simulink library "simetranss"  (R2024b)
settings: Solver=VariableStepAuto  StartTime=0.0  StopTime=10.0  RelTol=1e-3
PostLoadFcn:
  | Ts=1e-6
InitFcn:
  | Ts=1e-6
undefined symbols (not defined in the file): C, C_601, C_603, C_606, CC, Csnu, Csnubber, DiscIntNeverNeededParam, DPL, DPL1ph, FluxTable, ft2km, gcbh, h, Half, Imap2, L, L_601, L_603, L_606, Lbase, LpejoSw, Newton, R_601, R_603, R_606, Raphson, ResistanceM, Roff, Ron, RotorAngles, Rsnu, Rsnubber, Rt4, SampleTime, simetran, sps, sps_rtmsupport, StatorCurrents, T_2wind_ratio, T_Lpu, T_Lpu_pri, T_Rpu, T_Rpu_pri, T_Vpri, T_Vpri_15comp, T_Vsec, Ti, Ts_Power, Z, Zbase, Zm
libraries: fl_lib x248, ee_lib x146, nesl_utility x122, $bdroot x29, simulink x15, eeGeneralControl x2, spsStairGeneratorLib x2, artemis x1
(part 3 of 12)

== system simetranss/Network decoupling ==
  note: DC bus decoupling blocks
  DCbus Vrecv : Subsystem  mask(DC Bus decoupling (Receiving-V)){Ts=Ts}
      mask prompts: Ts "Sample time (s)"
      mask help: This block is used to create a delay in DC-busses..
      mask Display: disp('Vcap recv')
  DCbus Vsend : Subsystem  mask(DC Bus decoupling (Sending-V)){Ts=Ts}
      mask prompts: Ts "Sample time (s)"
      mask help: This block is used to create a delay in DC-busses.
      mask Display: disp('Vcap send')
  MATE 3-phase Compensated Half-Stubline : Subsystem  mask(MATE 3-phase Compensated Stubline){stype=3-phase line without couplings, FF=60, RR=R_601, LL=L_601, CC=C_601, len=2000*ft2km, Ts=Ts, comp=on, stdel=off}
      mask prompts: stype "Stubline type"; FF "Nominal frequency (Hz)"; RR "Resistance (Ohms/km)"; LL "Inductance (H/km)"; CC "Capacitance (F/km)"; len "Length (km)"; Ts "Sample time (s)"; comp "Compensate reactive power on this half of the stubline"; stdel "Concurrent simulation: remove internal stubline delay"
      mask help:
      | This block Implements a 3-phase stubline with reactive power compensation.
      |
      |
      | The block has 3 main options:
      | -uncoupled 3-phase
      | -single-mode coupled 3-phase
      | - dual-mode coupled 3-phase
      |
      | In single-mode, the stubline implements Bergeron line model with losses having the same 1-step propagation delay for all 3 modes. In the dual-mode option, the gound mode has a exact 2-step delay (main mode still has a 1 step-delay).The advantage of coupled modes is that some inter-phase capacitance is included in the stubline, therefore requirinf less overall reactive compensation.
      |
      | Line reactive compensation can only be made on only ONE of the two half stubline.
      |
      | Concurrent simulation: remove internal stubline delay : when using Simulink Concurrent simulation option, selecting this option removes the model 1/z communication delay, which is replaced implicitely by the concurrent simulation delay.
      mask init:
      | % Get current block
      | currentBlock = gcb;
      | 
      | dee=get_param(currentBlock,'stdel');
      | if isequal(dee,'on')
      |     set_param([currentBlock '/stubline/halfstub/zz'],'Commented','through');
      | else
      |     set_param([currentBlock '/stubline/halfstub/zz'],'Commented','off');
      | end
      | 
      | %Ts=2.5e-5;
      | % C1= (Ts)^2/L1;
      | Length=1;
      | Phases=3;
      | Frequency=FF;
      | Rabc = RR*len;
      | Labc = LL*len;
      | Cabc = CC*len;
      | 
      | Lm_abc_min = min(min(Labc));
      | Ls_abc_min = min(diag(Labc));
      | Lm_abc_max = max(max(Labc-diag(diag(Labc))));
      | 
      | Rm_abc_min = min(min(Rabc));
      | Rs_abc_min = min(diag(Rabc));
      | Rm_abc_max = max(max(Rabc-diag(diag(Rabc))));
      | 
      | Step = Ls_abc_min/10;
      | StepR = Rs_abc_min/10;
      | 
      | % xqnum=str2num(get_param(currentBlock,'xq'));
      | % x=xqnum(1);
      | % q=xqnum(2);
      | sel=0; % default delays all equal.
      | Ti=[1/sqrt(3) 1/sqrt(2)  1/sqrt(6); 1/sqrt(3) -1/sqrt(2)  1/sqrt(6); 1/sqrt(3) 0 -sqrt(2/3)];
      | st=get_param(currentBlock,'stype');
      | 
      | if isequal (st, '3-phase coupled line (1 mode)')
      |     %x=3
      |     %============== corrected code =====
      |     x=3;y=4;
      |     %===================================
      |     Lm = Lm_abc_min;
      |     L1 = 2*Lm;      %changed (is was L1 = 3*Lm;)
      |     Inductance = [x 1 1;1 x 1; 1 1 x]*L1/(x-1);
      |     L_diff = Labc - Inductance;
      | 
      |     Rm = Rm_abc_min;
      |     R1 = 2*Rm;      %changed (is was R1 = 3*Rm;)
      |     Resistance = [x 1 1;1 x 1; 1 1 x]*R1/(x-1);
      |     R_diff = Rabc - Resistance;
      | 
      | 
      |     if Ls_abc_min - 4*Lm - Step < Lm_abc_max - Lm
      |         Lm = (Ls_abc_min - Lm_abc_max - Step)/2;
      |         L1 = 2*Lm;      %changed (is was L1 = 3*Lm;)
      |         Inductance = [x 1 1;1 x 1; 1 1 x]*L1/(x-1);
      |         L_diff = Labc - Inductance;
      | 
      |         Rm = (Rs_abc_min - Rm_abc_max - StepR)/2;
      |         R1 = 2*Rm;      %changed (is was R1 = 3*Rm;)
      |         Resistance = [x 1 1;1 x 1; 1 1 x]*R1/(x-1);
      |         R_diff = Rabc - Resistance;
      |     end
      |     
      |     %=============== corrected code for capacitance =================
      |     C1 = Ts^2/L1;
      |     Capacitance =[y -1 -1;-1 y -1; -1 -1 y]*C1/(y+1);
      |     %==================================================================
      |     
      | 
      | elseif isequal(st,'3-phase coupled line (2 modes)')
      |     q=0.5;
      |     Lm = Lm_abc_min;
      |     L1 = Lm;
      |     Inductance = [1 q q; q 1 q; q q 1]*L1/(1-q);
      |     L_diff = Labc - Inductance; 
      | 
      |     R1 = Rm_abc_min ;
      |     Resistance = [1 q q; q 1 q; q q 1]*R1/(1-q);
      |     R_diff = Rabc - Resistance;
      | 
      |     Step = Ls_abc_min/10;
      |     StepR = Rs_abc_min/10;
      | 
      |     if Ls_abc_min - 2*Lm - Step < Lm_abc_max - Lm                                              
      |         Lm = Ls_abc_min - Lm_abc_max - Step;
      |         L1 = Lm;
      |         Inductance = [1 q q; q 1 q; q q 1]*L1/(1-q);
      |         L_diff = Labc - Inductance;
      | 
      |         R1 = Rs_abc_min - Rm_abc_max - StepR;
      |         Resistance = [1 q q; q 1 q; q q 1]*R1/(1-q);
      |         R_diff = Rabc - Resistance;
      |     end
      | 
      |     C1 = Ts^2/L1;
      |     Capacitance = eye(3)*C1; 
      |     
      | 
      | sel=1;  % with 2 mode case, mode 0 is 2 time slower!
      | 
      | elseif isequal(st,'3-phase line without couplings')
      |     L1 = Ls_abc_min - Lm_abc_max - Step;
      |     Inductance = eye(3)*L1;
      |     L_diff = Labc - Inductance;
      | 
      |     R1 = Rs_abc_min - Rm_abc_max - StepR;
      |     Resistance = eye(3)*R1;
      |     R_diff = Rabc - Resistance;
      |     C1 = Ts^2/L1;
      |     Capacitance = eye(3)*C1;   
      | else
      |     error('stubline type not found')
      | end
      | 
      | C_diff = Cabc;
      | 
      | % % Get electric variables
      | 
      | %============= These two lines should be removed ======
      | % C1 = Ts^2/L1
      | % Capacitance = eye(3)*C1;
      | %======================================================
      | 
      | [Zm,R,v,Ti,to,Rt4,h,Zimp,Zmat,Yphase,ResistanceM] = ssc_dpl_cb(currentBlock,'variable_mask_maskinitialization', Phases, Frequency, Resistance, Inductance, Capacitance, Length);
      | 
      | verif=sum(to/Ts);
      | if (2.99999<verif && verif<3.00001) || (3.99999<verif && verif<4.00001)
      |     % sum of delays should be 3 or 4
      | else
      |     error(['The stubline block ' gcb ' computed a non-integer propagation delay.']);
      | end
      | 
      | if isequal(st,'3-phase line without couplings')
      |     for i=1:3
      |         for j=1:3
      |             if i~=j  && ResistanceM(i,j)<0
      |                 ResistanceM(i,j)=1e10;   
      |             end
      |         end
      |     end
      | end
      | 
      | 
      | % % Compute Compensation block parameters
      | 
      | % Disabled here
      | 
      | L_comp=1/((2*pi*FF)^2*C1);     % calculate compensating inductance
      | R_damp=1e8;                     % set damping resistance to high value
      | C_damp=1e-8;                   % set coupling capacitor to low value
      mask TypeOptions stype: 3-phase coupled line (1 mode) | 3-phase coupled line (2 modes) | 3-phase line without couplings
      mask Callback comp:
      | block=gcb;
      | st=get_param(block,'comp');
      | if isequal(st,'on')
      |     set_param([block '/Compensate'], 'Commented', 'off');
      |     set_param([block '/Pass'], 'Commented', 'on');
      | else
      |     set_param([block '/Compensate'], 'Commented', 'on');
      |     set_param([block '/Pass'], 'Commented', 'off');
      | end
      mask Display:
      | plot(0,0,100,100,[20,20,40,40,60,40,40,20,20,10]+10,[50,40,40,50,50,50,61,61,50,50],[23 32 23 32]+10,[52,52,42,42],[33 35]+10,[55 55],[37 37]+10,[57 53])
      | 
      | %disp([ 32 32 'Full STUB'])
  RTScapeHalfStub : Subsystem  mask(SimScape Stubline){Phases=2 with differential inputs, pu=on, L=100e-3, Lpu=0.03, R=0.05, Rpu=0.02, S_base=1e5, V_base=1000, F_base=60, Ts=Ts}
      mask prompts: Phases "Number of phases N"; pu "Per-Unit value specification"; L "Inductance (H)"; Lpu "Inductance (pu)"; R "Resistance (Ohms)"; Rpu "Resistance (pu)"; S_base "Nominal Power (VA)"; V_base "Nominal voltage (V)"; F_base "Nominal frequency (Hz)"; Ts "Sample time (s)"
      mask help:
      | The simScape Stubline block implements a single distributed parameters transmission line model with exactly one time step propagation delay. It is optimized for real-time simulation.
      |
      | The SimScape Stubline block permits the decoupling of state-space system equations of networks on both sides of the stubline.
      mask init:
      | currentBlock = gcb;
      | 
      | 
      | 
      | % if isempty(S_base*V_base*F_base*Ts) 
      | %     return
      | % end
      | 
      | % Calculate Per Units
      | 
      | I_base=S_base/V_base;
      | w_base=2*pi*F_base;
      | Z_base=V_base/I_base;
      | L_base=Z_base/w_base;
      | C_base=1/(Z_base*w_base);
      | if pu == 1
      |     L=Lpu*L_base;
      |     R=Rpu*Z_base;
      | end
      | C = (Ts)^2/L;
      | Cpu = C / C_base;
      | 
      | 
      | 
      | 
      | 
      | 
      | % Calculate internal variables
      | [C, Zm, Rt4, h, w1, Z] = stub_cb(currentBlock,'lick it', 1, L, R, Ts);
      mask Help: eval('fts2help(''stubline'');');
      mask TypeOptions Phases: 1 | 2 | 3 | 4 | 5 | 6 | 2 with differential inputs
      mask Callback pu:
      | % Set mask display
      | stub_cb(gcb,'maskinitialization',1);
      mask Display: disp(sprintf('Half stubline\nL=  %s  mH\nC=  %s  uF\nR=  %s \\Omega',num2str(L*1e3,4), num2str(C*1e6,4), num2str(R,4)),'texmode','on');
  Seven-winding Decoupling Transformer : Subsystem  Tag=PublishSubsystem  mask(MATE 7-winding stubline transformer){Vpri=T_Vpri/sqrt(3), RLpri=[T_Rpu_pri*Zbase T_Lpu_pri*Lbase], Vwdn=[ T_Vsec/sqrt(3) T_Vsec T_Vsec/sqrt(3)*T_Vpri_15comp T_Vsec/sqrt(3)*T_2wind_ratio*T_Vpri_15comp T_Vsec/sqrt(3)*T_Vpri_15comp T_Vsec/sqrt(3)*T_2wind_ratio*T_Vpri_15comp  ], Lwdn=[T_Lpu_pri   T_Lpu T_Lpu T_Lpu*T_Vpri_15comp  T_Lpu*T_2wind_ratio*T_Vpri_15comp T_Lpu*T_Vpri_15comp  T_Lpu*T_2wind_ratio*T_Vpri_15comp ]*Lbase, Rwdn=[     T_Rpu            T_Rpu    T_Rpu*T_Vpri_15comp T_Rpu*T_2wind_ratio*T_Vpri_15comp T_Rpu*T_Vpri_15comp T_Rpu*T_2wind_ratio*T_Vpri_15comp]*Zbase, Rearth=1e6, Ts=Ts}
      mask prompts: Vpri "Primary voltage (V)"; RLpri "Primary winding resistance (Ohms) and leakaege inductance (H)"; Vwdn "Secondary winding voltages"; Lwdn "Secondary winding leakeage inductance (H)"; Rwdn "Secondary winding resistance (Ohms)"; Rearth "Secondary resistance to earth (Ohms)"; Ts "Sample time (s)"
      mask help: This is a stubline transformer in which all secondary windings are decoupled with a 1 step-delay transmission line (stubline).
  Three-Phase 2-Windings Decoupling Transformer : Subsystem  mask(MATE Decoupling Three-Phase Transformer (Two Windings)){deconf=Complete transformer, stdel=off, Winding1Connection=Yn, Winding2Connection=Yn, UNITS=pu, NominalPower=[ 500e3 , 60 ], Winding1=[ 4160 , 0.001 , 0.01 ], Winding2=[ 480, 0.01 , 0.01 ], Rm=500, Lm=500}
      mask prompts: deconf "Decoupling configuration"; stdel "Concurrent simulation: remove internal stubline delay"; Winding1Connection "Primary connection (ABC terminals):"; Winding2Connection "Secondary connection (abc terminals):"; NominalPower "Nominal power and frequency  [ Pn(VA) , fn(Hz) ]"; Winding1 "Winding 1 parameters [ V1 Ph-Ph(Vrms) , R1(pu) , L1(pu) ]"; Winding2 "Winding 2 parameters [ V2 Ph-Ph(Vrms) , R2(pu) , L2(pu) ]"; Rm "Magnetization resistance  Rm (pu)"; Lm "Magnetization inductance  Lm (pu)"
      mask help:
      | This block implements a  decoupling three-phase transformer.
      | The secondary winding leakeage inductance and resistance are implemented as stublines.
      | Only Y-Y with accesible neutral is available for now.
      mask init:
      | block = gcb;
      | dee=get_param(block,'stdel');
      | if isequal(dee,'on')
      |     set_param([block '/del1'],'Commented','through');
      |     set_param([block '/del2'],'Commented','through');
      |     set_param([block '/del3'],'Commented','through');
      |     set_param([block '/del4'],'Commented','through');
      | else
      |     set_param([block '/del1'],'Commented','off');
      |     set_param([block '/del2'],'Commented','off');
      |     set_param([block '/del3'],'Commented','off');
      |     set_param([block '/del4'],'Commented','off');
      | end
      | 
      | m=ThreePhaseTransformersPU(block);
      | 
      | block = gcb;
      | str=get_param(block,'deconf');
      | if isequal(str,'Complete transformer')
      |     set_param([block '/pri'], 'Commented', 'off');
      |     set_param([block '/sec'], 'Commented', 'off');
      |     set_param([block '/path'], 'Value', '1');
      |     replace_block (block ,'Followlinks' ,'on' ,'Name' ,'houtsec' ,'BlockType' ,'Outport' ,'Terminator' ,'noprompt' );
      |     replace_block (block ,'Followlinks' ,'on' ,'Name' ,'houtpri' ,'BlockType' ,'Outport' ,'Terminator' ,'noprompt' );
      |     replace_block (block ,'Followlinks' ,'on' ,'Name' ,'hinsec' ,'BlockType' ,'Inport' ,'Ground' ,'noprompt' );
      |     replace_block (block ,'Followlinks' ,'on' ,'Name' ,'hinpri' ,'BlockType' ,'Inport' ,'Ground' ,'noprompt' );
      |     MATE_xfo_ports(block, 'addABC');
      |     MATE_xfo_ports(block, 'addN');
      |     MATE_xfo_ports(block, 'addabc');
      |     MATE_xfo_ports(block, 'addn');
      | elseif isequal(str,'Primary side')
      |     set_param([block '/pri'], 'Commented', 'off');
      |     set_param([block '/sec'], 'Commented', 'on');
      |     set_param([block '/path'], 'Value', '0');
      |     try
      |     replace_block (block ,'Followlinks' ,'on' ,'Name' ,'houtsec' ,'BlockType' ,'Outport' ,'Terminator' ,'noprompt' );
      |     replace_block (block ,'Followlinks' ,'on' ,'Name' ,'houtpri' ,'BlockType' ,'Terminator','Outport' ,'noprompt' );
      |     replace_block (block ,'Followlinks' ,'on' ,'Name' ,'hinsec' ,'BlockType' ,'Inport' ,'Ground' ,'noprompt' );
      |     replace_block (block ,'Followlinks' ,'on' ,'Name' ,'hinpri' ,'BlockType' ,'Ground' ,'Inport' ,'noprompt' );
      |     catch
      |         warning('possible port error on Primary')
      |     end
      |     MATE_xfo_ports(block, 'addABC');
      |     MATE_xfo_ports(block, 'addN');
      |     MATE_xfo_ports(block, 'removeabc');
      |     MATE_xfo_ports(block, 'removen');
      | elseif isequal(str,'Secondary side')
      |     set_param([block '/pri'], 'Commented', 'on');
      |     set_param([block '/sec'], 'Commented', 'off');
      |     set_param([block '/path'], 'Value', '0');
      |     try
      |     replace_block (block ,'Followlinks' ,'on' ,'Name' ,'houtsec' ,'BlockType' ,'Terminator','Outport' ,'noprompt' );
      |     replace_block (block ,'Followlinks' ,'on' ,'Name' ,'houtpri' ,'BlockType' ,'Outport' ,'Terminator','noprompt' );
      |     replace_block (block ,'Followlinks' ,'on' ,'Name' ,'hinsec' ,'BlockType' , 'Ground' ,'Inport','noprompt' );
      |     replace_block (block ,'Followlinks' ,'on' ,'Name' ,'hinpri' ,'BlockType' ,'Inport' ,'Ground' ,'noprompt' );
      |     catch
      |         warning('possible port error on Secondary')
      |     end
      |     MATE_xfo_ports(block, 'removeABC');
      |     MATE_xfo_ports(block, 'removeN');
      |     MATE_xfo_ports(block, 'addabc');
      |     MATE_xfo_ports(block, 'addn');
      | else 
      |     error('Option not reckognized!')
      | end
      mask TypeOptions deconf: Complete transformer | Primary side | Secondary side
      mask TypeOptions Winding1Connection: Y | Yn | Yg | Delta (D1) | Delta (D11)
      mask TypeOptions Winding2Connection: Y | Yn | Yg | Delta (D1) | Delta (D11)
      mask TypeOptions UNITS: SI | pu
      mask DialogControl ParameterTabVar0 Prompt: Configuration
      mask DialogControl ParameterTabVar01 Prompt: Parameters
      mask Display:
      | plot(-180,-220,180,220,[-100,-40],[0,0],[100,40],[0,0],[2 42 74 94 100 90 66 30 0 2 42 74 94 100 90 66 30 0 2 42 74 94 100 90 66 30 0 2 42 74 94 100 90 66 30 0]*.4-55,[-45 -45 -34 -17 3 22 38 48 50 50 55 66 83 103 122 138 148 150 150 155 166 183 203 222 238 248 250 250 255 266 283 303 322 338 348 348]*0.5-75,[2 42 74 94 100 90 66 30 0 2 42 74 94 100 90 66 30 0 2 42 74 94 100 90 66 30 0 2 42 74 94 100 90 66 30 0]*-.4+55,[-45 -45 -34 -17 3 22 38 48 50 50 55 66 83 103 122 138 148 150 150 155 166 183 203 222 238 248 250 250 255 266 283 303 322 338 348 348]*0.5-75)
      | %plot(-180,-220,180,220,[-100,-40]*-1,[0,0],[2 42 74 94 100 90 66 30 0 2 42 74 94 100 90 66 30 0 2 42 74 94 100 90 66 30 0 2 42 74 94 100 90 66 30 0]*.4-55,[-45 -45 -34 -17 3 22 38 48 50 50 55 66 83 103 122 138 148 150 150 155 166 183 203 222 238 248 250 250 255 266 283 303 322 338 348 348]*-0.5+75)
      | 
      | disp(['Y   Y'  10 10 10 10 10 'z-1'])
  wires:
  DCbus Vsend/1(Vc) -> DCbus Vrecv/1(Vc-z)
  DCbus Vrecv/1(Idc) -> DCbus Vsend/1(Iin)

== system simetranss/Passive ==
  MATE Single-Phase Load : Subsystem  mask(MATE 1-phase load){Vabc=300, Fn=60, typ=Series RL, Pabc=[160 ]*1e3, QLabc=[ 90]*1e3, QCabc=[190  ]*1e3}
      mask prompts: Vabc "Nominal phase-to-ground voltage (Vrms)"; Fn "Nominal frequency fn (Hz):"; typ "Load type"; Pabc "Active powers (W)"; QLabc "Inductive reactive powers (positive var):"; QCabc "Capacitive reactive powers (positive var):"
      mask help: This block implements either a series RL load or a purely capacitive load.
      mask init:
      | block=gcb;
      | type=get_param(block,'typ');
      | 
      | if isequal (type,'Series RL')
      | j=sqrt(-1);
      | S=Pabc-j*QLabc;
      | Z=Vabc.*Vabc./S;
      | R=real(Z);
      | L=imag(Z)/2/pi/Fn;
      | 
      | s1 = 0;
      | s2 =-50;
      | s3 = 450;
      | s4 =50;
      | r1 = [0    30    30    38    53    68    83    98   113   120   120   150];
      | r2 =[0     0     0    25   -25    25   -25    25   -25     0     0     0];
      | c1 =[0];
      | c2 =[0 ];
      | c3 =[0];
      | c4 = [0];
      | c5=0;
      | c6=0;
      | l1 =[150   173   173   174   178   184   190   197   202   205   206   204   201 201   197   196   198   201   207   214   220   225   229   229   227   224   224   220   219   221   225   230   237   243   249   252   253   251   247  247   244   243   244   248   254   260   267   272   275   276   276   300 450];
      | l2 =[0     0     1    11    19    24    25    23    17     8    -2   -12   -18 -18    -9     1    11    19    24    25    23    17     8    -2   -12   -18 -18    -9     1    11    19    24    25    23    17     8    -2   -12   -18  -18    -9     1    11    19    24    25    23    17     8     0     0     0 0];
      | sca=0.5;
      | neutral=0;
      | ground=1;
      | else
      |     j=sqrt(-1);
      | S=QCabc;
      | Z=Vabc.*Vabc./S;
      | w=2*pi*Fn;
      | % Z=1/(wC)
      | C=1/w./Z;
      | 
      | 
      | s1 = 0;
      | s2 =-50;
      | s3 = 450;
      | s4 =50;
      | r1 = [0    ];
      | r2 =[0   ];
      | c1 =[450   390   390   393   395   393   390   390   393   395]-200;
      | c2 =[0     0     8    16    25    16     8    -8   -16   -25];
      | c3 =[360   360   360   250]-200;
      | c4 = [25   -25     0     0];
      | c5 =[ 455 200];
      | c6 = [0 0];
      | l1 =[0];
      | l2 =[0 ];
      | sca=0.5;
      | neutral=0;
      | 
      | ground=1;
      | 
      | 
      | 
      | end
      mask TypeOptions typ: Series RL | Capacitance
      mask Callback typ:
      | block = gcb;
      | type=get_param(block,'typ');
      | 
      | visib=get_param(block,'MaskVisibilities');
      | if isequal(type,'Series RL')
      |     visib{4}='on';;visib{5}='on';visib{6}='off';
      | else
      |     visib{4}='off';visib{5}='off';visib{6}='on';
      | end
      | set_param(block,'MaskVisibilities',visib);
      | 
      | 
      | if isequal(type,'Series RL')
      |     set_param([block '/RLseries'], 'Commented', 'off');
      |     set_param([block '/C'], 'Commented', 'on');
      | else
      |     set_param([block '/RLseries'], 'Commented', 'on');
      |     set_param([block '/C'], 'Commented', 'off');
      | end
      mask Display:
      | plot(s1-160,s2,s3+80,s4,r1,r2,l1,l2,c1,c2,c3,c4,c5,c6)
      | 
      | plot( ground*[s3,s3], ground*[-s2/4,s2/4])
      | plot( ground*[s3+30,s3+30], ground*[-s2/6,s2/6])
      | plot( ground*[s3+60,s3+60], ground*[-s2/10,s2/10])
      | 
      | plot( neutral*[s3,s3+80], neutral*[0,0])
  MATE Unbalanced Load : Subsystem  AncestorBlock=simetran/SimScape RL Load3  mask(MATE  3-phase unbalanced load){Vabc=[ 0.993926 1.02168 0.995885]*277.128, Fn=60, typ=Series RL, Pabc=[160 120 120]*1e3, QLabc=[110 90 90]*1e3, QCabc=[190  60  212]*1e3}
      mask prompts: Vabc "Nominal phase-to-neutral voltages [Va Vb Vc] (Vrms)"; Fn "Nominal frequency fn (Hz):"; typ "Load type"; Pabc "Active powers [Pa Pb Pc] (W):"; QLabc "Inductive reactive powers [QLa QLb QLc] (positive var):"; QCabc "Capacitive reactive powers [QCa QCb QCc] (positive var):"
      mask help: This block implements either a series RL load or a purely capacitive load.
      mask init: same as simetranss/Passive/MATE Single-Phase Load
      mask TypeOptions typ: Series RL | Capacitance
      mask Callback typ:
      | block = gcb;
      | type=get_param(block,'typ');
      | 
      | visib=get_param(block,'MaskVisibilities');
      | if isequal(type,'Series RL')
      |     visib{4}='on';;visib{5}='on';visib{6}='off';
      | else
      |     visib{4}='off';visib{5}='off';visib{6}='on';
      | end
      | set_param(block,'MaskVisibilities',visib);
      | 
      | 
      | if isequal(type,'Series RL')
      |     set_param([block '/RLseries'], 'Commented', 'off');
      |     set_param([block '/C'], 'Commented', 'on');
      | else
      |     set_param([block '/RLseries'], 'Commented', 'on');
      |     set_param([block '/C'], 'Commented', 'off');
      | end
      mask Display:
      | disp(['                      3ph'  10])
      | plot(s1-160,s2,s3+80,s4,r1,r2,l1,l2,c1,c2,c3,c4,c5,c6)
      | 
      | plot( ground*[s3,s3], ground*[-s2/4,s2/4])
      | plot( ground*[s3+30,s3+30], ground*[-s2/6,s2/6])
      | plot( ground*[s3+60,s3+60], ground*[-s2/10,s2/10])
      | 
      | plot( neutral*[s3,s3+80], neutral*[0,0])
  MATE Unbalanced LoadDEV1 : Subsystem  mask(MATE  3-phase unbalanced load){yd=Delta, Vabc=[ 0.993926 1.02168 0.995885]*277.128, VabcDelta=[ 1 1 1]*277.128, Fn=60, typ=Series RL, Pabc=[160 120 120]*1e3, QLabc=[110 90 90]*1e3, QCabc=[190  60  212]*1e3}
      mask prompts: yd "Configuration"; Vabc "Nominal phase-to-ground voltages [Va Vb Vc] (Vrms)"; VabcDelta "Nominal phase-to-phase voltage [Vab Vbc Vca] (Vrms)"; Fn "Nominal frequency fn (Hz):"; typ "Load type"; Pabc "Active powers [Pa Pb Pc] (W):"; QLabc "Inductive reactive powers [QLa QLb QLc] (positive var):"; QCabc "Capacitive reactive powers [QCa QCb QCc] (positive var):"
      mask help: This block implements either a series RL load or a purely capacitive load.
      mask init:
      | block=gcb;
      | type=get_param(block,'typ');
      | conf=get_param(block,'yd');
      | 
      | if isequal (type,'Series RL')
      | j=sqrt(-1);
      | S=Pabc-j*QLabc;
      | Z=Vabc.*Vabc./S;
      | R=real(Z);
      | L=imag(Z)/2/pi/Fn;
      | 
      | s1 = 0;
      | s2 =-50;
      | s3 = 450;
      | s4 =50;
      | r1 = [0    30    30    38    53    68    83    98   113   120   120   150];
      | r2 =[0     0     0    25   -25    25   -25    25   -25     0     0     0];
      | c1 =[0];
      | c2 =[0 ];
      | c3 =[0];
      | c4 = [0];
      | c5=0;
      | c6=0;
      | l1 =[150   173   173   174   178   184   190   197   202   205   206   204   201 201   197   196   198   201   207   214   220   225   229   229   227   224   224   220   219   221   225   230   237   243   249   252   253   251   247  247   244   243   244   248   254   260   267   272   275   276   276   300 450];
      | l2 =[0     0     1    11    19    24    25    23    17     8    -2   -12   -18 -18    -9     1    11    19    24    25    23    17     8    -2   -12   -18 -18    -9     1    11    19    24    25    23    17     8    -2   -12   -18  -18    -9     1    11    19    24    25    23    17     8     0     0     0 0];
      | sca=0.5;
      | neutral=0;
      | ground=1;
      | else
      |     j=sqrt(-1);
      | S=QCabc;
      | Z=Vabc.*Vabc./S;
      | w=2*pi*Fn;
      | % Z=1/(wC)
      | C=1/w./Z;
      | 
      | 
      | s1 = 0;
      | s2 =-50;
      | s3 = 450;
      | s4 =50;
      | r1 = [0    ];
      | r2 =[0   ];
      | c1 =[450   390   390   393   395   393   390   390   393   395]-200;
      | c2 =[0     0     8    16    25    16     8    -8   -16   -25];
      | c3 =[360   360   360   250]-200;
      | c4 = [25   -25     0     0];
      | c5 =[ 455 200];
      | c6 = [0 0];
      | l1 =[0];
      | l2 =[0 ];
      | sca=0.5;
      | neutral=0;
      | 
      | ground=1;
      | 
      | 
      | 
      | end
      mask TypeOptions yd: Grounded Y | Delta
      mask Callback yd:
      | block = gcb;
      | type=get_param(block,'yd');
      | 
      | visib=get_param(block,'MaskVisibilities');
      | if isequal(type,'Grounded Y')
      |     visib{2}='on';visib{3}='off';
      | else
      |     visib{2}='off';visib{3}='on';
      | end
      | set_param(block,'MaskVisibilities',visib);
      mask TypeOptions typ: Series RL | Capacitance
      mask Callback typ:
      | block = gcb;
      | type=get_param(block,'typ');
      | 
      | visib=get_param(block,'MaskVisibilities');
      | if isequal(type,'Series RL')
      |     visib{6}='on';;visib{7}='on';visib{8}='off';
      | else
      |     visib{6}='off';visib{7}='off';visib{8}='on';
      | end
      | set_param(block,'MaskVisibilities',visib);
      | 
      | 
      | if isequal(type,'Series RL')
      |     set_param([block '/RLseries'], 'Commented', 'off');
      |     set_param([block '/C'], 'Commented', 'on');
      | else
      |     set_param([block '/RLseries'], 'Commented', 'on');
      |     set_param([block '/C'], 'Commented', 'off');
      | end
      mask Display:
      | disp(['                      3ph'  10])
      | plot(s1-160,s2,s3+80,s4,r1,r2,l1,l2,c1,c2,c3,c4,c5,c6)
      | 
      | plot( ground*[s3,s3], ground*[-s2/4,s2/4])
      | plot( ground*[s3+30,s3+30], ground*[-s2/6,s2/6])
      | plot( ground*[s3+60,s3+60], ground*[-s2/10,s2/10])
      | 
      | plot( neutral*[s3,s3+80], neutral*[0,0])
  RLC : Subsystem  mask(SimScape Electrical single-phase RLC Branch){BranchType=RL, SerPar=Parallel, Resistance=1, Inductance=1e-3, Capacitance=1e-6, Ropen=1e9}
      mask prompts: BranchType "Branch type:"; SerPar "Branch type:"; Resistance "Resistance (Ohms):"; Inductance "Inductance (H):"; Capacitance "Capacitance (F):"; Ropen "Open-circuit resistance (Ohms)"
      mask help:
      | Implements a series/parallel branch of RLC elements in single-phase.
      |
      | Models the resistive, capacitive, and inductive characteristics of a three-phase line. You can represent the impedance of each of the three lines as either a series or a parallel combination of a resistor, capacitor, and inductor.
      mask init:
      | block=gcb;
      | if isequal(get_param(block,'SerPar'),'Series')
      |     x1=0;x2=0;x3=0;x4=0;
      | [s1,s2,s3,s4,r1,r2,l1,l2,c1,c2,c3,c4] = MATEdrawRLC('Series RLC Branch',Resistance,Inductance,Capacitance,BranchType);
      | else
      | [s1,s2,s3,s4,r1,r2,l1,l2,c1,c2,c3,c4,x1,x2,x3,x4] = MATEdrawRLC('Parallel RLC Branch',Resistance,Inductance,Capacitance,BranchType);
      | end
      | 
      | BranchType =get_param (block ,'BranchType' ); 
      | 
      | MaskVisibilities ={'on' ,'on' ,'off' ,'off' ,'off','off'};
      | 
      | if strfind(BranchType,'R')
      |     MaskVisibilities{3}='on';
      | end
      | if strfind(BranchType,'L')
      |     MaskVisibilities{4}='on';
      | end
      | if strfind(BranchType,'C')
      |     MaskVisibilities{5}='on';
      | end
      | if strfind(BranchType,'O')
      |     MaskVisibilities{6}='on';
      | end
      | set_param (block ,'MaskVisibilities' ,MaskVisibilities ); 
      | 
      | Resistance2=Resistance;
      | show=[1 1 1 1 1 1 1];
      | name={
      |     'R'
      |     'L'
      |     'C'
      |     'RLCs_1'
      |     'RLCs_2'
      |     'RLCp_1'
      |     'RLCp_2'
      |     };
      | switch BranchType
      |     case 'R'
      |         show=[1 0 0 0 0 0 0];
      |     case 'L'
      |         show=[0 1 0 0 0 0 0];
      |     case 'C'
      |         show=[0 0 1 0 0 0 0];
      |     case 'RL'
      |         if SerPar==1
      |             show=[0 1 0 0 0 0 0];
      |         else
      |             Resistance2=0;
      |             show=[1 1 0 0 0 0 0];
      |         end
      |     case 'RC'
      |          if SerPar==1
      |             show=[0 0 1 0 0 0 0];
      |          else
      |             Resistance2=0; 
      |             show=[1 0 1 0 0 0 0];
      |          end
      |     case 'LC'
      |         Resistance2=0;
      |         if SerPar==1
      |             show=[0 0 0 1 1 0 0];
      |         else
      |             show=[0 0 0 0 0 1 1];
      |         end
      |     case 'RLC'
      |         if SerPar==1
      |             show=[0 0 0 1 1 0 0];
      |         else
      |             show=[0 0 0 0 0 1 1];
      |         end
      |      case 'Open circuit'
      |         typn=1;
      |         Resistance=Ropen;
      |         show=[1 0 0 0 0 0 0];
      |         
      |     otherwise
      |         error('Error RLC branch selection')
      | end
      | 
      | for i=1:7
      |     if show(i)==1
      |         set_param([block '/' name{i} ],'Commented','off');
      |     else
      |         set_param([block '/' name{i} ],'Commented','on');
      |     end
      | end
      mask TypeOptions BranchType: RLC | R | L | C | RL | RC | LC | Open circuit
      mask TypeOptions SerPar: Series | Parallel
      mask Display:
      | %plot(s1,s2,s3,s4,r1,r2*1.5,l1,l2*1.5,c1,c2*1.5,c3,c4*1.5)
      | plot(s1,s2,s3,s4,r1,r2,l1,l2,c1,c2,c3,c4,x1,x2,x3,x4);
      | color('blue')
      | port_label('LConn',1,'+')
  RLC(3ph) : Subsystem  mask(SimScape Electrical 3-phase RLC Branch){BranchType=RLC, SerPar=Series, Resistance=1, Inductance=1e-3, Capacitance=1e-6, Ropen=1e9}
      mask prompts: BranchType "Branch type:"; SerPar "Branch type:"; Resistance "Resistance (Ohms):"; Inductance "Inductance (H):"; Capacitance "Capacitance (F):"; Ropen "Open-circuit resistance (Ohms)"
      mask help:
      | Implements a series/parallel branch of RLC elements.
      |
      | Models the resistive, capacitive, and inductive characteristics of a three-phase line. You can represent the impedance of each of the three lines as either a series or a parallel combination of a resistor, capacitor, and inductor.
      mask init:
      | block=gcb;
      | if isequal(get_param(block,'SerPar'),'Series')
      |     x1=0;x2=0;x3=0;x4=0;
      | [s1,s2,s3,s4,r1,r2,l1,l2,c1,c2,c3,c4] = MATEdrawRLC('Series RLC Branch',Resistance,Inductance,Capacitance,BranchType);
      | else
      | [s1,s2,s3,s4,r1,r2,l1,l2,c1,c2,c3,c4,x1,x2,x3,x4] = MATEdrawRLC('Parallel RLC Branch',Resistance,Inductance,Capacitance,BranchType);
      | end
      | 
      | BranchType =get_param (block ,'BranchType' ); 
      | 
      | MaskVisibilities ={'on' ,'on' ,'off' ,'off' ,'off','off'};
      | 
      | if strfind(BranchType,'R')
      |     MaskVisibilities{3}='on';
      | end
      | if strfind(BranchType,'L')
      |     MaskVisibilities{4}='on';
      | end
      | if strfind(BranchType,'C')
      |     MaskVisibilities{5}='on';
      | end
      | if strfind(BranchType,'O')
      |     MaskVisibilities{6}='on';
      | end
      | set_param (block ,'MaskVisibilities' ,MaskVisibilities ); 
      | 
      | typ={
      | 'ee.enum.rlc.structure.R'
      | 'ee.enum.rlc.structure.L'
      | 'ee.enum.rlc.structure.C'
      | 'ee.enum.rlc.structure.SeriesRL'
      | 'ee.enum.rlc.structure.SeriesRC'
      | 'ee.enum.rlc.structure.SeriesLC'
      | 'ee.enum.rlc.structure.SeriesRLC'
      | 'ee.enum.rlc.structure.ParallelRL'
      | 'ee.enum.rlc.structure.ParallelRC'
      | 'ee.enum.rlc.structure.ParallelLC'
      | 'ee.enum.rlc.structure.ParallelRLC'
      | };
      | 
      | switch BranchType
      |     case 'R'
      |         typn=1;
      |     case 'L'
      |         typn=2;
      |     case 'C'
      |         typn=3;
      |     case 'RL'
      |         if SerPar==1
      |             typn=4;
      |         else
      |             typn=8;
      |         end
      |     case 'RC'
      |          if SerPar==1
      |             typn=5;
      |         else
      |             typn=9;
      |          end
      |     case 'LC'
      |         if SerPar==1
      |             typn=6;
      |         else
      |             typn=10;
      |         end
      |     case 'RLC'
      |         if SerPar==1
      |             typn=7;
      |         else
      |             typn=11;
      |         end
      |      case 'Open circuit'
      |         typn=1;
      |         Resistance=Ropen;
      |         
      |     otherwise
      |         error('Error RLC branch selection')
      | end
      | 
      | set_param([block '/RLC3'],'component_structure',typ{typn})
      mask TypeOptions BranchType: RLC | R | L | C | RL | RC | LC | Open circuit
      mask TypeOptions SerPar: Series | Parallel
      mask Display:
      | %plot(s1,s2,s3,s4,r1,r2*1.5,l1,l2*1.5,c1,c2*1.5,c3,c4*1.5)
      | plot(s1,s2,s3,s4,r1,r2,l1,l2,c1,c2,c3,c4,x1,x2,x3,x4);
      | color('blue')
      | port_label('LConn',1,'+')
      | disp(['3ph'  10 10])

== system simetranss/Power converters ==
  MATE_3LevelNPCinverter : Subsystem  mask(MATE 3-level NPC inverter){Arms=1, SnubberResistance=Rsnu, SnubberCapacitance=Csnu, Device=IGBT / Diodes, Ron=1e-3, Vf=1, ihiz=999}
      mask prompts: Arms "Number of bridge arms:"; SnubberResistance "Snubber resistance Rs (Ohms)"; SnubberCapacitance "Snubber capacitance Cs (F)"; Device "Power Electronic device (IGBT, GTO,MOSFET are equivalent)"; Ron "Internal resistance Ron (Ohms)"; Vf "Forward Device voltage  (V)"; ihiz "High Impedance current tolerance"
      mask help:
      | MATE Three-Level Inverter
      |
      | This model implements a 3-level NPC inverter using a surrogate circuit.
      | The surrogate circuit has only 3 switches and associated RC snubber.
      | The 3 switches connects the output phase connection A to each of inputs of inverter(V+, N, V-) and are controlled using an algorithm that mimics the behavior of real 3-level NPC inverters.
      |
      | Parameters:
      |
      | Snubber resistance Rs (Ohms): Resistance of the RC-snubber.
      | Snubber capacitance Cs (F): Capacitance of the RC snubber.
      | Internal resistance Ron (Ohms): Conduction resistance of all switches.
      |
      | Gate signal (size 4). Drive the 4 IGBTs from the + rail to neutral rail, to the - rail in this order.
      mask init:
      | X.p1= [39 39 23.8000];
      |     X.p2= [44 56 49.6000 56 52.8000 56 61 61];
      |     X.p3= [44 44 44 61 61];
      |     X.p4= [75 67 83 75 67 83 75 75];
      |     X.p5= [61 75 75];
      |     X.p6= [75 75 61];
      |     X.p7= 0;
      | 
      |     Y.p1= [71 28 28];
      |     Y.p2= [  39.2000   33.6000   32.8000   33.6000   40.8000   33.6000  30.0000   12.4000];
      |     Y.p3= [28 71 60 66.4000 90];
      |     Y.p4= [54 42 42 54 54 54 54 66];
      |     Y.p5= [24 24 42];
      |     Y.p6= [66 76 76];
      |     Y.p7= 0;
      mask TypeOptions Arms: 1
      mask TypeOptions Device: IGBT / Diodes
  MATE_3LevelNPCinverter(3ph) : Subsystem
  MATE_Cascaded_Hbridge_Inverter : Subsystem  mask(MATE H-Bridge Multi-Level Converter){Gtype=Mean Active Duty (0<=g<=1), nbc=4, ron=0.001, roff=1e5, Ts=Ts}
      mask prompts: Gtype "Gating type"; nbc "Number of stages"; ron "IGBT Ron (Ohms)"; roff "IGBT Roff (Ohms)"; Ts "Sample Time (s)"
      mask help:
      | This model implements a cascaded H-bridge multi-level converter. Underneath is a nodal admittance solver.
      |
      | Gate order: From upper level H-bridge to lower ones.
      | Each H-bridge order is left arm, upper and lower IGBTs, right arm, upper and lower IGBTs.
      |
      | When connected to oversampling blocks or FPGA, the model can be fed with Mean Active Duty for each IGBTs, that is the per-unit value of ON-time per time step.
      mask init:
      | bloc=gcb;
      | 
      | 
      | 
      | 
      | % Digital (g=0 or g=1)
      | % Mean Active Duty (0<=g<=1)
      | 
      | ttyp=get_param(bloc,'Gtype');
      | if isequal(ttyp, 'Digital (g=0 or g=1)')
      |     gt=1;
      | elseif isequal(ttyp, 'Mean Active Duty (0<=g<=1)')
      |     gt=2;
      | else
      |     error;
      | end
      mask TypeOptions Gtype: Digital (g=0 or g=1) | Mean Active Duty (0<=g<=1)
  MATE_MMCarm : Subsystem  mask(SimScape MMC module (half-bridge)){nbc=200, ron=Ron, roff=Roff, cc=CC, Ts=Ts, rf=on, dts=on}
      mask prompts: nbc "Number of cell"; ron "IGBT Ron (Ohms)"; roff "IGBT Roff (Ohms)"; cc "Cell capacitance (F)"; Ts "Sample Time (s)"; rf "Non-infinite Roff"; dts "Disabled time stamping"
      mask help:
      | This model implements an half-bridge MMC module with full nodal solution, i.e. there is no delay between the MMC and then main solver solution and the MMC module is seen as a discrete Thevenin equivalent to the main Simscape solver.
      |
      | This is a detailed model with each module having a distinct capacitor voltage.
      |
      | g: all upper IGBT gates (the lower ones are generated internally)
      | blk: block the pulse when =1
      | Vc: all capacitor voltage
      mask init:
      | for k=1:4
      |     switch k
      |          case 1
      |               R1=roff; R2=roff;
      |               A(k)=0; B(k)=0; C(k)=0; D(k)=R2;
      |          case 2
      |               R1=ron; R2=roff;
      |               A(k)=0; B(k)=1/cc; C(k)=1; D(k)=R1;
      |          case 3
      |               R1=roff; R2=ron;
      |               A(k)=0; B(k)=0; C(k)=0; D(k)=R2;
      |          case 4
      |              R1=ron; R2=ron;
      |              A(k)=0; B(k)=0; C(k)=0; D(k)=R2; %incorrect but not supposed to happen
      |     end
      |     if isequal(get_param(gcb,'rf'),'on')
      |      rr=(1+R2/R1);
      |      A(k)=-1/R1/cc/rr;
      |      B(k)=R2/R1/cc/rr;
      |      C(k)=R2/R1/rr;
      |      D(k)=R2/rr;
      |     end
      |          
      |        %% choose here if you want trapeze or backward Euler (more stable) 
      |         if 1==0 % trap
      |             Ad(k) = (1-Ts/2*A(k))\(1+Ts/2*A(k));         %SS discretize
      |             Bd1(k) = (1-Ts/2*A(k))\(Ts/2*B(k));    %SS discretize
      |             Bd2(k) = (1-Ts/2*A(k))\(Ts/2*B(k));    %SS discretize
      |         else % BE
      |             Ad(k) = 1/(1-Ts*A(k));         %SS discretize
      |             Bd2(k) = Ts*B(k)/(1-Ts*A(k));    %SS discretize
      |             Bd1(k) =0;
      |         end
      |         Z(k)=C(k)'.*Bd2(k) + D(k);
      | end
      | 
      | 
      | dtsval=1; %must be = 1
  Oversampled Switching function 2-level IGBT/diode inverter (3ph) : Subsystem  mask(Switching Function 2-level inverter(3ph)){Ron=1e-3, Rsnubber=100, Csnubber=1e-6, Vf=1, Ts=Ts_Power}
      mask prompts: Ron "Switch conduction resistance (Ohms)"; Rsnubber "Snubber resistance (Ohms)"; Csnubber "Snubber capacitance (F)"; Vf "Diode forward voltage (V)"; Ts "Sample Time (s)"
      mask help:
      | This block implements a 2-level inverter as a swtiching function with high-impedance capability.
      |
      | With proper Time-Step Averaged duty cycle at the gate inputs, this model can accurately simulation PWM modulation with deadtimes smaller than the simulation time step.
      settings: CopyFcn=%set_param(gcb,'LinkStatus','inactive');
  Switching Function Interpolating 2-level inverter : Subsystem  mask(Inverter Switching Function (2-level IGBT/Diode)){Ron=Ron, Gp=Rsnubber, Gi=Csnubber, Ts=Ts, dc_short_resistance=0.1}
      mask prompts: Ron "Switch Ron [Ohms]"; Gp "Snubber resistance [Ohms]"; Gi "Snubber Capacitor [Farads]"; Ts "Sample time [s]"; dc_short_resistance "Anti-parallel diode resistance (Ohms)"
      mask help: This block implements a 2-level inverter as a switching function.

== system simetranss/Switches ==
  MATE 3ph Breaker : Subsystem  mask(MATE Three-Phase Breaker){InitialState=open, SwitchA=on, SwitchB=on, SwitchC=off, SwitchTimes=[1/60  5/60], External=off, BreakerResistance=0.01, Roff=1e6, SnubberResistance=1e6, SnubberCapacitance=inf}
      mask prompts: InitialState "Initial status:"; SwitchA "Phase A"; SwitchB "Phase B"; SwitchC "Phase C"; SwitchTimes "Switching times (s):"; BreakerResistance "Breaker resistance Ron (Ohm):"; Roff "Breaker resistance Roff (Ohms)"; SnubberResistance "Snubber resistance Rs (Ohm):"; SnubberCapacitance "Snubber capacitance Cs (F):"
      mask help:
      | Implements a three-phase circuit breaker. When the external switching time mode is selected, a Simulink logical signal is used to control the breaker operation.
      |
      | This breaker is ON when the gate value =1 and OFF when the gate value=0.
      mask init:
      | block = gcb;
      | [X ,Y ,SwitchStates ,InitialState ,Switch_Times ]=MATEBreakerInit(block,InitialState,SwitchTimes,External,SnubberResistance,SnubberCapacitance);
      | MaskEnables =get_param (block ,'MaskEnables' ); 
      | 
      | if strcmp (get_param (block ,'External' ),'on' )
      | MaskEnables {5 }='off' ; 
      | else
      | MaskEnables {5 }='on' ; 
      | end
      | 
      | MaskEnables {7 }='on' ; 
      |  
      | MaskEnables {8 }='on' ; 
      | MaskEnables {9 }='on' ; 
      | 
      | set_param (block ,'MaskEnables' ,MaskEnables ); 
      | 
      | X.p1=-20;
      | X.p2=120;
      | 
      | if SnubberCapacitance>1e8
      |     set_param([block '/RCsnubber'], 'Commented', 'on');
      | else
      |     set_param([block '/RCsnubber'], 'Commented', 'off');
      | end
      mask TypeOptions InitialState: open | closed
      mask DialogControl Container3 Prompt: Switching of:
      mask Display: plot(X.p1,Y.p1,X.p2,Y.p2,X.p3,Y.p3,X.p4,Y.p4,X.p5,Y.p5,X.p6,Y.p6)
  MATE Breaker : Subsystem  mask(MATE Single-Phase Breaker){InitialState=open, SwitchA=on, SwitchB=on, SwitchC=off, SwitchTimes=[1/60  5/60], External=off, BreakerResistance=0.01, Roff=1e6, SnubberResistance=1e6, SnubberCapacitance=inf}
      mask prompts: InitialState "Initial status:"; SwitchA "Phase A"; SwitchB "Phase B"; SwitchC "Phase C"; SwitchTimes "Switching times (s):"; BreakerResistance "Breaker resistance Ron (Ohm):"; Roff "Breaker resistance Roff (Ohms)"; SnubberResistance "Snubber resistance Rs (Ohm):"; SnubberCapacitance "Snubber capacitance Cs (F):"
      mask help:
      | Implements a single-phase circuit breaker. When the external switching time mode is selected, a Simulink logical signal is used to control the breaker operation.
      |
      | This breaker is ON when the gate value =1 and OFF when the gate value=0.
      mask init: same as simetranss/Switches/MATE 3ph Breaker
      mask TypeOptions InitialState: open | closed
      mask DialogControl Container3 Prompt: Switching of:
      mask Display: plot(X.p1,Y.p1,X.p2,Y.p2,X.p3,Y.p3,X.p4,Y.p4,X.p5,Y.p5,X.p6,Y.p6)

== system simetranss/Usefulls ==
  Event Timer : Subsystem  Tag=RTEcontrol_s38shd7k88  LoadFcn=|  mask(Timer){is=0 (off), t=[0.01 0.02 0.03 0.04 ], Tmax=0.07, Ts=Ts}
      | xx=get_param(gcb,'linkstatus');      
      | if isequal(xx,'inactive')            
      | set_param(gcb,'linkstatus','restore')
      | end
      mask prompts: is "Initial state"; t "Transition times (s):"; Tmax "Repeat period (s)"; Ts "Sample time (s)"
      mask help: This block generates a Simulink control signal changing at specified transition times.
      mask init:
      | iss=get_param(gcb,'is');
      | if isequal(iss,'0 (off)')
      |     sw(1)=0;
      |     sw(2)=0;
      | else
      |     sw(1)=1;
      |     sw(2)=1;
      | end
      | st(1)=0;
      | st(2)=t(1);
      | 
      | if t(1)==0,
      |    h=errordlg(' The first time specified must be greater than 0 ' , 'Parameter error');
      | end
      | 
      | i=3;
      | tog=0;
      | ptr=2;
      | while length(sw)<=2*length(t)
      |     if tog==0
      |         st=[st st(end)+Ts];
      |         sw=[sw 1-sw(end)];
      |         tog=1;
      |     else
      |         st=[st t(ptr)];
      |         sw=[sw sw(end)];
      |         ptr=ptr+1;
      |         tog=0;
      |     end
      | 
      | end
      |  %st=[st Tmax-Ts Tmax+Ts]
      | % sw=[sw sw(end) sw(1)]
      mask TypeOptions is: 0 (off) | 1 (on)
      mask Display:
      | %plot(0,0,100,100,[70,40,40,20,20,13],[30,30,70,70,30,30]);
      | plot( st(1:end-1), sw(1:end-1) );
  ModelInitialization : Subsystem  mask(Model Initialisation){InitFcnX=Ts=1e-6, prel=off, posl=on, inif=on, strf=off}
      mask prompts: InitFcnX "Initialisation"; prel "Preload Function"; posl "PostLoad Function"; inif "InitFcn"; strf "StartFcn"
      mask help: This block sets the model Initialisation function conviniently.
      mask init:
      | if prel==1
      | 	set_param(bdroot, 'PreLoadFcn', InitFcnX);
      | else
      | 	set_param(bdroot, 'PreLoadFcn', '');
      | end
      | if inif==1
      | 	set_param(bdroot, 'InitFcn', InitFcnX);
      | else
      | 	set_param(bdroot, 'InitFcn', '');
      | end
      | if strf==1
      | 	set_param(bdroot, 'StartFcn', InitFcnX);
      | else
      | 	set_param(bdroot, 'StartFcn', '');
      | end
      | if posl==1
      | 	set_param(bdroot, 'PostLoadFcn', InitFcnX);
      | else
      | 	set_param(bdroot, 'PostLoadFcn', '');
      | end
      | PLF = get_param(bdroot, 'PreLoadFcn');
      | IF = get_param(bdroot, 'InitFcn');
      | SF = get_param(bdroot, 'StartFcn');
      | 
      | 
      | pos = get_param(gcb, 'Position');
      | width = pos(3) - pos(1); height = pos(4) - pos(2);
      mask Display:
      | text(5, height*0.5, [ ...
      |   ...
      | '  '  get_param(bdroot, 'InitFcn')  ...
      | ], ...
      | 'horizontalAlignment', 'left', 'verticalAlignment', 'middle') ;

== system simetranss/FPGA/MATE 2-level inverter ==
  gate : Inport
  Demux2 : Demux  Outputs=2
  lower : $bdroot/FPGA/Pejovic L-C-switch component  typ=2-level inverter switch  Lon=Lon  L=L  C=C  otherSW='coming soon'  Ts=Ts
  upper : $bdroot/FPGA/Pejovic L-C-switch component  typ=2-level inverter switch  Lon=Lon  L=L  C=C  otherSW='coming soon'  Ts=Ts
  V+ : PMIOPort  Side=Left
  Vout : PMIOPort  Port=2  Side=Right
  V- : PMIOPort  Port=3  Side=Left
  wires:
  lower/1 -> upper/2
  upper/1 -> lower/2
  gate/1 -> Demux2/1
  Demux2/1 -> upper/1
  Demux2/2 -> lower/1
  connections:
  lower/RConn1 -- V-/RConn1
  upper/LConn1 -- V+/RConn1
  lower/LConn1 -- Vout/RConn1 -- upper/RConn1
